simulink model "wheel_odometry"  (R2023a)
settings: Solver=FixedStepAuto  StartTime=0.0  StopTime=inf  FixedStep=0.01  RelTol=1e-3
model workspace (MAT data in the model file):
  L = 2.66
  R = 0.347
  Tw = 1.565
  b = 1.61
  k = 1
undefined symbols (not defined in the file): pose, twist
libraries: ros2lib x6, simulink x1
settings Model: SimulationMode=external  Creator=roma  LastModifiedBy=roma
settings DataIOCC: ReturnWorkspaceOutputs=off
settings OptimizationCC: EnhancedBackFolding=on  PassReuseOutputArgsAs=Individual arguments  ZeroExternalMemoryAtStartup=off  ZeroInternalMemoryAtStartup=off  MaxStackSize=64  OptimizeBlockOrder=speed  DifferentSizesBufferReuse=on  OptimizationCustomize=off  EfficientTunableParamExpr=on
settings DebuggingCC: ParameterTunabilityLossMsg=error
settings HardwareCC: ProdBitPerLong=64  ProdHWDeviceType=Intel->x86-64 (Linux 64)
settings SFSimCC: MATLABDynamicMemAlloc=off
settings RTWCC: Description=Embedded Coder  SystemTargetFile=ert.tlc  HardwareBoard=Robot Operating System 2 (ROS 2)  TLCOptions="-aInlineSetEventsForThisBaseRateFcn=TLC_FALSE -aSuppressMultiTaskScheduler=TLC_FALSE  -aRateBasedStepFcn=0"  GenCodeOnly=on  TemplateMakefile=ert_default_tmf  Toolchain=Colcon Tools  TargetLang=C++
settings CodeAppCC: ForceParamTrailComments=on  IgnoreCustomStorageClasses=off  OperatorAnnotations=on  SimulinkDataObjDesc=on  SFDataObjDesc=on  InsertBlockDesc=on
settings ERTTargetCC: CodeInterfacePackaging=C++ class  SupportContinuousTime=on  RootIOFormat=Structure reference

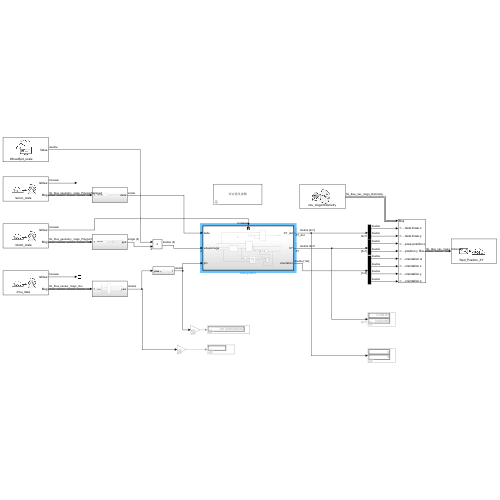
[thumbnail: Simulink's stored preview of the top-level diagram]
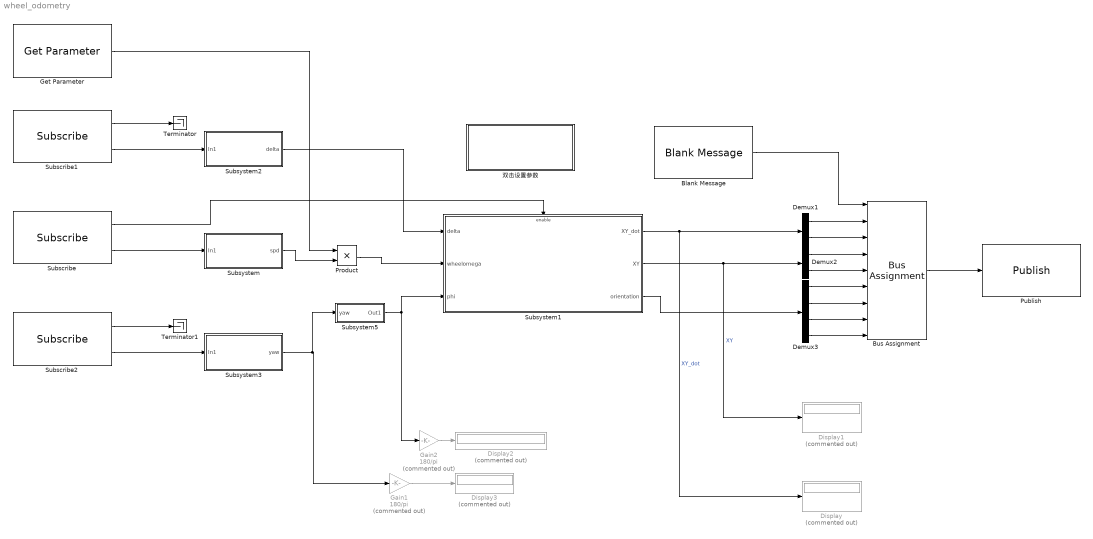
== system wheel_odometry ==
  Blank Message : ros2lib/Blank Message  messageClass=Message  entityType=nav_msgs/Odometry  messageType=nav_msgs/Odometry  SampleTime=-1
  Bus Assignment : BusAssignment  AssignedSignals=twist.twist.linear.x,twist.twist.linear.y,pose.pose.position.x,pose.pose.position.y,pose.pose.orientation.w,pose.pose.orientation.x,pose.pose.orientation.y,pose.pose.orientation.z
  Demux1 : Demux  Outputs=2
  Demux2 : Demux  Outputs=2
  Demux3 : Demux
  Display{,1..3} (4 alike) : Display  Commented=on
  Gain1 : Gain  Commented=on  Gain=180/pi
  Gain2 : Gain  Commented=on  Gain=180/pi
  Get Parameter : ros2lib/Get Parameter  ParameterName=WheelSpd_scale  ParameterType=double  ParameterMaxArrayLength=16  ParameterInitialValue=1  SampleTime=-1  ModelName=wheel_odometry  BlockId=ParamGet_wheel_odometry_353
  Product : Product
  Publish : ros2lib/Publish  topicSource=Specify your own  topic=/Spd_Position_XY  messageType=nav_msgs/Odometry  QOSHistory=Keep last  QOSDepth=1  QOSReliability=Best effort  QOSDurability=Volatile
  Subscribe : ros2lib/Subscribe  topicSource=Select from ROS network  topic=/motor_state  messageType=geometry_msgs/PolygonStamped  sampleTime=0.01  QOSHistory=Keep last  QOSDepth=1  QOSReliability=Best effort  QOSDurability=Volatile
  Subscribe1 : ros2lib/Subscribe  topicSource=Select from ROS network  topic=/servo_state  messageType=geometry_msgs/PolygonStamped  sampleTime=0.01  QOSHistory=Keep last  QOSDepth=1  QOSReliability=Reliable  QOSDurability=Volatile
  Subscribe2 : ros2lib/Subscribe  topicSource=Select from ROS network  topic=/Imu_data  messageType=sensor_msgs/Imu  sampleTime=0.01  QOSHistory=Keep last  QOSDepth=1  QOSReliability=Best effort  QOSDurability=Volatile
  Subsystem : Subsystem
  Subsystem1 : Subsystem
  Subsystem2 : Subsystem
  Subsystem3 : Subsystem
  Subsystem5 : Subsystem
  Terminator : Terminator
  Terminator1 : Terminator
  双击设置参数 : Subsystem  mask{k=1, R=0.347, b=1.61, L=2.66, Tw=1.565}
      mask init:
      | % hws = get_param(gcs, 'modelworkspace');
      |     % temp = double(string(get_param(gcb,'k')));
      |     % hws.assignin('k', temp);
      |     % temp = double(string(get_param(gcb,'R')));
      |     % hws.assignin('R', temp);
      |     % temp = double(string(get_param(gcb,'b')));
      |     % hws.assignin('b', temp);
      |     % temp = double(string(get_param(gcb,'L')));
      |     % hws.assignin('L', temp);
      |     % % clear temp hws R b L
      mask Callback k:
      | hws = get_param(gcs, 'modelworkspace');
      |     temp = double(string(get_param(gcb,'k')));
      |     hws.assignin('k', temp);
      |     clear temp hws
      mask Callback R:
      | hws = get_param(gcs, 'modelworkspace');
      |     temp = double(string(get_param(gcb,'R')));
      |     hws.assignin('R', temp);
      |     clear temp hws
      mask Callback b:
      | hws = get_param(gcs, 'modelworkspace');
      |     temp = double(string(get_param(gcb,'b')));
      |     hws.assignin('b', temp);
      |     clear temp hws
      mask Callback L:
      | hws = get_param(gcs, 'modelworkspace');
      |     temp = double(string(get_param(gcb,'L')));
      |     hws.assignin('L', temp);
      |     clear temp hws
      mask Callback Tw:
      | hws = get_param(gcs, 'modelworkspace');
      |     temp = double(string(get_param(gcb,'Tw')));
      |     hws.assignin('Tw', temp);
      |     clear temp hws
      mask DialogControl Control2 Prompt: 设置初始工况
      mask Display: disp('双击更改参数');
  wires:
  Subsystem1/1(XY_dot) -> Display/1, Demux1/1  "XY_dot"
  Subsystem1/2(XY) -> Display1/1, Demux2/1  "XY"
  Subscribe/2 -> Subsystem/1(In1)
  Subsystem/1(spd) -> Product/2
  Subscribe1/2 -> Subsystem2/1(In1)
  Subsystem2/1(delta) -> Subsystem1/1(delta)
  Subscribe2/2 -> Subsystem3/1(In1)
  Subscribe1/1 -> Terminator/1
  Subscribe2/1 -> Terminator1/1
  Subscribe/1 -> Subsystem1/Enable
  Blank Message/1 -> Bus Assignment/1
  Bus Assignment/1 -> Publish/1
  Demux1/1 -> Bus Assignment/2
  Demux1/2 -> Bus Assignment/3
  Demux2/1 -> Bus Assignment/4
  Demux2/2 -> Bus Assignment/5
  Product/1 -> Subsystem1/2(wheelomega)
  Subsystem3/1(yaw) -> Subsystem5/1(yaw), Gain1/1
  Gain1/1 -> Display3/1
  Gain2/1 -> Display2/1
  Subsystem5/1(Out1) -> Gain2/1, Subsystem1/3(phi)
  Get Parameter/1 -> Product/1
  Subsystem1/3(orientation) -> Demux3/1
  Demux3/1 -> Bus Assignment/6
  Demux3/2 -> Bus Assignment/7
  Demux3/3 -> Bus Assignment/8
  Demux3/4 -> Bus Assignment/9

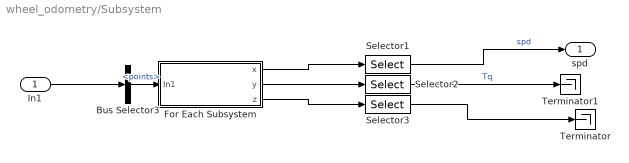
== system wheel_odometry/Subsystem ==
  In1 : Inport
  Bus Selector3 : BusSelector  OutputSignals=polygon.points
  For Each Subsystem : Subsystem  TreatAsAtomicUnit=on
  Selector1 : Selector  InputPortWidth=16  IndexOptions=Index vector (dialog)  Indices=[1:4]  OutputSizes=1
  Selector2 : Selector  InputPortWidth=16  IndexOptions=Index vector (dialog)  Indices=[1:4]  OutputSizes=1
  Selector3 : Selector  InputPortWidth=16  IndexOptions=Index vector (dialog)  Indices=[1:4]  OutputSizes=1
  Terminator : Terminator
  Terminator1 : Terminator
  spd : Outport
  wires:
  For Each Subsystem/2(y) -> Selector2/1
  Selector3/1 -> Terminator/1
  For Each Subsystem/3(z) -> Selector3/1
  For Each Subsystem/1(x) -> Selector1/1
  Bus Selector3/1 -> For Each Subsystem/1(In1)  "<points>"
  Selector1/1 -> spd/1  "spd"
  In1/1 -> Bus Selector3/1
  Selector2/1 -> Terminator1/1  "Tq"

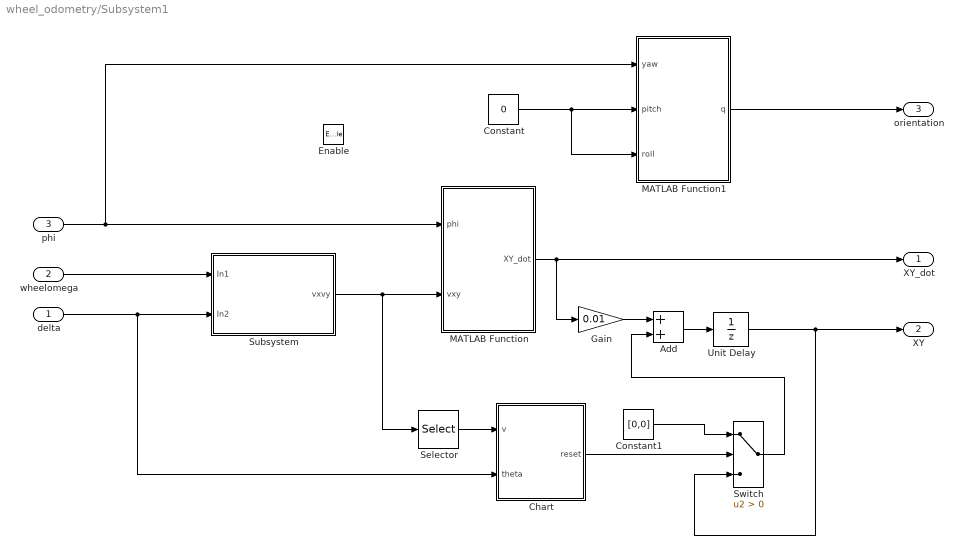
== system wheel_odometry/Subsystem1 ==
  delta : Inport
  wheelomega : Inport  Port=2
  phi : Inport  Port=3
  Enable : EnablePort
  Add : Sum
  Chart : Stateflow chart  TreatAsAtomicUnit=on
  Constant : Constant  Value=0
  Constant1 : Constant  Value=[0,0]
  Gain : Gain  Gain=0.01
  MATLAB Function : MATLAB Function  TreatAsAtomicUnit=on
  MATLAB Function1 : MATLAB Function  TreatAsAtomicUnit=on
  Selector : Selector  InputPortWidth=2  IndexOptions=Index vector (dialog)  Indices=[1]  OutputSizes=1
  Subsystem : Subsystem
  Switch : Switch  Criteria=u2 > Threshold  SaturateOnIntegerOverflow=off  InputSameDT=off
  Unit Delay : UnitDelay  SampleTime=-1  HasFrameUpgradeWarning=on
  XY_dot : Outport
  XY : Outport  Port=2
  orientation : Outport  Port=3
  wires:
  wheelomega/1 -> Subsystem/1(In1)
  delta/1 -> Chart/2(theta), Subsystem/2(In2)
  phi/1 -> MATLAB Function1/1(yaw), MATLAB Function/1(phi)
  MATLAB Function/1(XY_dot) -> Gain/1, XY_dot/1
  Unit Delay/1 -> Switch/3, XY/1
  Gain/1 -> Add/1
  Add/1 -> Unit Delay/1
  Constant/1 -> MATLAB Function1/3(roll), MATLAB Function1/2(pitch)
  MATLAB Function1/1(q) -> orientation/1
  Chart/1(reset) -> Switch/2
  Selector/1 -> Chart/1(v)
  Subsystem/1(vxvy) -> MATLAB Function/2(vxy), Selector/1
  Constant1/1 -> Switch/1
  Switch/1 -> Add/2

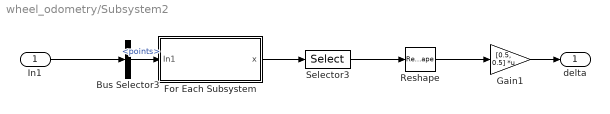
== system wheel_odometry/Subsystem2 ==
  In1 : Inport
  Bus Selector3 : BusSelector  OutputSignals=polygon.points
  For Each Subsystem : Subsystem  TreatAsAtomicUnit=on
  Gain1 : Gain  Gain=[0.5, 0.5]  Multiplication=Matrix(K*u)
  Reshape : Reshape  OutputDimensionality=Column vector (2-D)
  Selector3 : Selector  InputPortWidth=16  IndexOptions=Index vector (dialog)  Indices=[1:2]  OutputSizes=1
  delta : Outport
  wires:
  In1/1 -> Bus Selector3/1
  Bus Selector3/1 -> For Each Subsystem/1(In1)  "<points>"
  For Each Subsystem/1(x) -> Selector3/1
  Selector3/1 -> Reshape/1
  Reshape/1 -> Gain1/1
  Gain1/1 -> delta/1

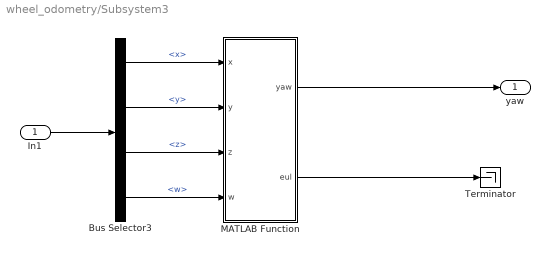
== system wheel_odometry/Subsystem3 ==
  In1 : Inport
  Bus Selector3 : BusSelector  OutputSignals=orientation.x,orientation.y,orientation.z,orientation.w
  MATLAB Function : MATLAB Function  TreatAsAtomicUnit=on
  Terminator : Terminator
  yaw : Outport
  wires:
  In1/1 -> Bus Selector3/1
  MATLAB Function/1(yaw) -> yaw/1
  MATLAB Function/2(eul) -> Terminator/1
  Bus Selector3/1 -> MATLAB Function/1(x)  "<x>"
  Bus Selector3/2 -> MATLAB Function/2(y)  "<y>"
  Bus Selector3/3 -> MATLAB Function/3(z)  "<z>"
  Bus Selector3/4 -> MATLAB Function/4(w)  "<w>"

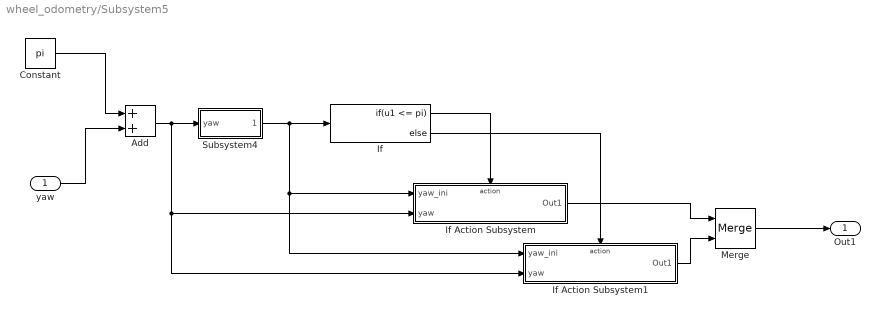
== system wheel_odometry/Subsystem5 ==
  yaw : Inport
  Add : Sum
  Constant : Constant  Value=pi
  If : If  IfExpression=u1 <= pi
  If Action Subsystem : Subsystem  TreatAsAtomicUnit=on
  If Action Subsystem1 : Subsystem  TreatAsAtomicUnit=on
  Merge : Merge
  Subsystem4 : Subsystem
  Out1 : Outport
  wires:
  yaw/1 -> Add/2
  Constant/1 -> Add/1
  Add/1 -> If Action Subsystem1/2(yaw), If Action Subsystem/2(yaw), Subsystem4/1(yaw)
  If/1 -> If Action Subsystem/Action
  If/2 -> If Action Subsystem1/Action
  If Action Subsystem/1(Out1) -> Merge/1
  If Action Subsystem1/1(Out1) -> Merge/2
  Merge/1 -> Out1/1
  Subsystem4/1(yaw_ini) -> If Action Subsystem1/1(yaw_ini), If Action Subsystem/1(yaw_ini), If/1

== system wheel_odometry/双击设置参数 ==

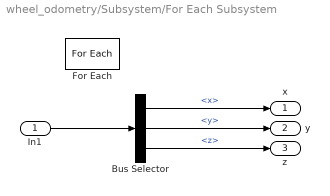
== system wheel_odometry/Subsystem/For Each Subsystem ==
  In1 : Inport  Partition=on  PartitionDimension=1  PartitionWidth=1  PartitionOffset=0
  Bus Selector : BusSelector  OutputSignals=x,y,z
  For Each : ForEach  DisableCoverage=on
  x : Outport  ConcatenationDimension=1
  y : Outport  Port=2  ConcatenationDimension=1
  z : Outport  Port=3  ConcatenationDimension=1
  wires:
  In1/1 -> Bus Selector/1
  Bus Selector/1 -> x/1  "<x>"
  Bus Selector/2 -> y/1  "<y>"
  Bus Selector/3 -> z/1  "<z>"

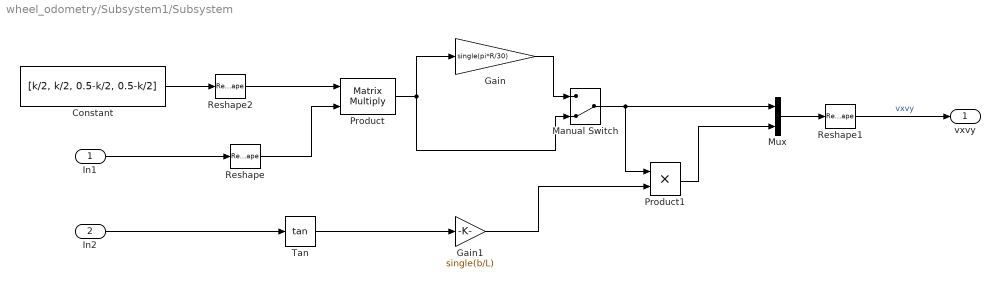
== system wheel_odometry/Subsystem1/Subsystem ==
  In1 : Inport  PortDimensions=[4,1]
  In2 : Inport  Port=2
  Constant : Constant  Value=[k/2, k/2, 0.5-k/2, 0.5-k/2]
  Gain : Gain  Gain=single(pi*R/30)
  Gain1 : Gain  Gain=single(b/L)
  Manual Switch : ManualSwitch  CurrentSetting=0
  Mux : Mux  Inputs=2
  Product : Product  Multiplication=Matrix(*)
  Product1 : Product
  Reshape : Reshape  OutputDimensionality=Column vector (2-D)
  Reshape1 : Reshape  OutputDimensionality=Column vector (2-D)
  Reshape2 : Reshape  OutputDimensionality=Row vector (2-D)
  Tan : Trigonometry  Operator=tan
  vxvy : Outport
  wires:
  Product1/1 -> Mux/2
  Gain1/1 -> Product1/2
  Mux/1 -> Reshape1/1
  Constant/1 -> Reshape2/1
  Tan/1 -> Gain1/1
  Product/1 -> Gain/1, Manual Switch/2
  Manual Switch/1 -> Mux/1, Product1/1
  Reshape/1 -> Product/2
  In2/1 -> Tan/1
  In1/1 -> Reshape/1
  Reshape1/1 -> vxvy/1  "vxvy"
  Reshape2/1 -> Product/1
  Gain/1 -> Manual Switch/1

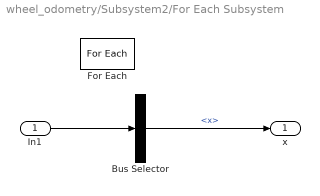
== system wheel_odometry/Subsystem2/For Each Subsystem ==
  In1 : Inport  Partition=on  PartitionDimension=1  PartitionWidth=1  PartitionOffset=0
  Bus Selector : BusSelector  OutputSignals=x
  For Each : ForEach  DisableCoverage=on
  x : Outport  ConcatenationDimension=1
  wires:
  Bus Selector/1 -> x/1  "<x>"
  In1/1 -> Bus Selector/1

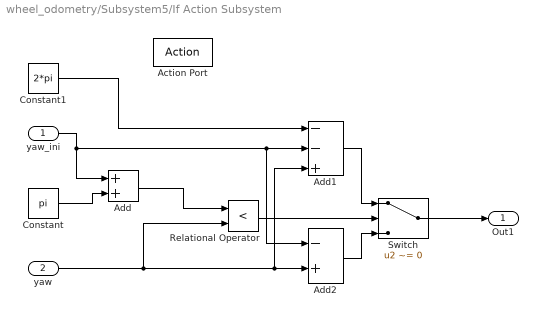
== system wheel_odometry/Subsystem5/If Action Subsystem ==
  yaw_ini : Inport
  yaw : Inport  Port=2
  Action Port : ActionPort  ActionPortLabel=if(u1 <= pi)
  Add : Sum
  Add1 : Sum  Inputs=--+
  Add2 : Sum  Inputs=-+
  Constant : Constant  Value=pi
  Constant1 : Constant  Value=2*pi
  Relational Operator : RelationalOperator  Operator=<  OutDataTypeStr=boolean  RndMeth=Simplest  InputSameDT=off
  Switch : Switch  Criteria=u2 ~= 0  SaturateOnIntegerOverflow=off  InputSameDT=off
  Out1 : Outport
  wires:
  Constant/1 -> Add/2
  Add/1 -> Relational Operator/1
  yaw/1 -> Relational Operator/2, Add1/3, Add2/2
  Relational Operator/1 -> Switch/2
  Constant1/1 -> Add1/1
  Add1/1 -> Switch/1
  Switch/1 -> Out1/1
  yaw_ini/1 -> Add/1, Add2/1, Add1/2
  Add2/1 -> Switch/3

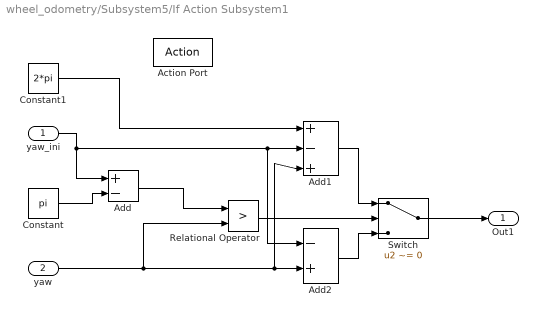
== system wheel_odometry/Subsystem5/If Action Subsystem1 ==
  yaw_ini : Inport
  yaw : Inport  Port=2
  Action Port : ActionPort  ActionPortLabel=else
  Add : Sum  Inputs=+-
  Add1 : Sum  Inputs=+-+
  Add2 : Sum  Inputs=-+
  Constant : Constant  Value=pi
  Constant1 : Constant  Value=2*pi
  Relational Operator : RelationalOperator  Operator=>  OutDataTypeStr=boolean  RndMeth=Simplest  InputSameDT=off
  Switch : Switch  Criteria=u2 ~= 0  SaturateOnIntegerOverflow=off  InputSameDT=off
  Out1 : Outport
  wires:
  Switch/1 -> Out1/1
  Add1/1 -> Switch/1
  Constant1/1 -> Add1/1
  Relational Operator/1 -> Switch/2
  yaw/1 -> Add1/3, Add2/2, Relational Operator/2
  Add/1 -> Relational Operator/1
  Constant/1 -> Add/2
  yaw_ini/1 -> Add2/1, Add1/2, Add/1
  Add2/1 -> Switch/3

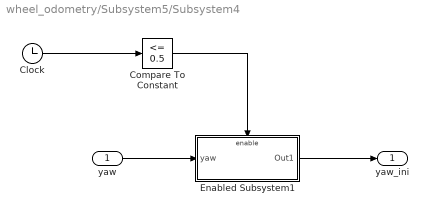
== system wheel_odometry/Subsystem5/Subsystem4 ==
  yaw : Inport
  Clock : Clock
      settings: Decimation=2
  Compare To Constant : simulink/Logic and Bit Operations/Compare To Constant  relop=<=  const=0.5  OutDataTypeStr=boolean
  Enabled Subsystem1 : Subsystem  TreatAsAtomicUnit=on
  yaw_ini : Outport
  wires:
  Enabled Subsystem1/1(Out1) -> yaw_ini/1
  Clock/1 -> Compare To Constant/1
  Compare To Constant/1 -> Enabled Subsystem1/Enable
  yaw/1 -> Enabled Subsystem1/1(yaw)

== system wheel_odometry/Subsystem5/Subsystem4/Enabled Subsystem1 ==
  yaw : Inport
  Enable : EnablePort
  Out1 : Outport
  wires:
  yaw/1 -> Out1/1

== matlab function wheel_odometry/Subsystem3/MATLAB Function ==
  data: x input; yaw output; y input; z input; w input; eul output
function [yaw, eul] = fcn(x, y, z, w)

yaw = atan2(2*(w*z+x*y),1-2*(y^2+z^2));
% roll = atan2(2*(w*x+y*z),1-2*(x^2+y^2));
% pitch = asin(2*(w*y-z*x));
% q = [x, y, z, w];
% eul = quat2eul(q);% w,x,y,z
eul = 0;

== matlab function wheel_odometry/Subsystem1/MATLAB Function ==
  data: phi input; XY_dot output; vxy input
function XY_dot = fcn(phi, vxy)

R = [cos(phi),-sin(phi);sin(phi),cos(phi)];
XY_dot = R*vxy;

== matlab function wheel_odometry/Subsystem1/MATLAB Function1 ==
  data: yaw input; q output; pitch input; roll input
function q = fcn(yaw, pitch, roll)

q = eul2quat([yaw,pitch,roll]);

== stateflow chart wheel_odometry/Subsystem1/Chart ==
  state hold
    en,du:
    reset = false;
  state clearXY
    en:
    reset = true;
    delay = int16(5);
    du:
    delay = delay-int16(1);
  state waiting
  state waiting1
  (default) -> hold
  hold -> waiting [order 1] : [abs(v)<0.01 && theta>0.6]
  waiting -> clearXY [order 1] : [theta<-0.6]
  waiting -> hold [order 2] : [abs(v) >=0.1]
  clearXY -> hold : [delay<int16(2)]
  hold -> waiting1 [order 2] : [abs(v)<0.01 && theta<-0.6]
  waiting1 -> clearXY [order 2] : [theta>0.6]
  waiting1 -> hold [order 1] : [abs(v) >=0.1]
  data: v input; theta input; delay local int16; reset output int8
